simulink model "hoppingControl"  (R2018b)
settings: Solver=FixedStepAuto  StartTime=0.0  StopTime=inf  RelTol=1e-3  EnableMultiTasking=on
libraries: dspstat3 x19, cm_custom x9, raspberrypilib x8, simulink_extras x3, peGeneralControl x3, can_bus_multi x2, simulink x1, embdlinuxlib x1
(part 2 of 3)

== matlab function hoppingControl/Joint Position Filter/MATLAB Function ==
  data: motor_pos input; bias output; set_offset input; corrected_pos output; safe output
function [bias,corrected_pos, safe] = correct_pos(motor_pos, set_offset)
persistent offset;
persistent safety;
if(isempty(safety))
    safety = -1;
end

if(isempty(offset))
    offset = [0; 0; 0];
end


bias = offset;
if(set_offset~=0)
    offset = motor_pos(1:3);
    safety = 0;
elseif safety == 0
    safety = 1;
end
corrected_pos = motor_pos(1:3)-offset;
for i = 1:3
    if(corrected_pos(i)>180)
        corrected_pos(i) = corrected_pos(i) - 360;
    end

    if(corrected_pos(i)<-180)
        corrected_pos(i) = corrected_pos(i) + 360;
    end
    corrected_pos(i) = corrected_pos(i)+90;
    if corrected_pos(i)>90
        corrected_pos(i) = 90;
    end
end





safe = safety;
end

== matlab function hoppingControl/state estimation/MATLAB Function ==
  data: velInc input; vel output; angVelInc input; angVel input; viconPos input; viconOrient input; velLambda input; orientLambda input; orient output; realAngVel output; vVel output; vOrient output size=[1 4]; viconTime input; orientReset input; vPos output
function [vel,orient,realAngVel,vVel,vOrient,vPos] = sensorFusion(velInc, angVelInc, angVel, viconPos, viconOrient, velLambda, ...
                                                                  orientLambda,viconTime, orientReset)
persistent lastOrient;
if isempty(lastOrient)
    lastOrient = quaternion(1,0,0,0);
end
persistent lastOrientTime;
if isempty(lastOrientTime)
    lastOrientTime = 0;
end
persistent lastViconQuat;
if isempty(lastViconQuat)
    lastViconQuat = quaternion(1,0,0,0);
end

imu2vicon = [0  0 -1; % rotation matrix of robot frame in vicon to imu frame
            -1  0  0;
             0  1  0];
quatInc = compact(quaternion((imu2vicon*angVelInc)','rotvec'));
if quatInc(1)<0
    quatInc = -quatInc;
end
quatInc = quaternion(quatInc);
temp = compact(lastOrient * quatInc);
if temp(1)<0
    temp = -temp;
end
lastOrient = quaternion(temp);
if abs(viconTime-lastOrientTime)>=0.01
    viconQuat = compact(quaternion(viconOrient','euler','XYZ','frame'));
    if viconQuat(1)<0
        viconQuat = -viconQuat;
    end
    viconQuat = quaternion(viconQuat);
    errorQuat = viconQuat*conj(lastOrient);
    errorQuat = compact(errorQuat);
    if errorQuat(1)<0
        errorQuat = -errorQuat;
    end
    errorAngle = asin(norm(errorQuat(2:4)))*2;
    correctAngle = orientLambda*errorAngle;
    correctQuat = compact(quaternion(correctAngle*errorQuat(2:4)/norm(errorQuat(2:4)),'rotvec'));
    if correctQuat(1)<0
        correctQuat = -correctQuat;
    end
    correctQuat = quaternion(correctQuat);
    lastOrient = (correctQuat)*lastOrient;
    lastOrientTime = viconTime;
    lastViconQuat = viconQuat;
end

persistent lastVel;
if isempty(lastVel)
    lastVel = [0;0;0];
end
persistent lastViconVel;
if isempty(lastViconVel)
    lastViconVel = [0;0;0];
end
persistent lastPos;
if isempty(lastPos)
    lastPos = [0;0;0];
end
persistent lastViconVel2;
if isempty(lastViconVel2)
    lastViconVel2 = [0;0;0];
end
persistent lastPos2;
if isempty(lastPos2)
    lastPos2 = [0;0;0];
end
persistent lastVelTime
if isempty(lastVelTime)
    lastVelTime = 0;
end
lastVel = lastVel - quat2rotm(lastOrient)*imu2vicon*velInc - [0;0;9.81]*0.002;
if abs(viconTime - lastVelTime)>=0.01
    pos = viconPos +  quat2rotm(lastViconQuat)*[-0.01388;0.02222;-0.1656]; % robot center from vicon object center in vicon frame
    lastViconVel = (pos - lastPos)/(viconTime-lastVelTime);
    lastPos = pos;
    
    pos2 = viconPos +  quat2rotm(lastViconQuat)*[-0.0291;0.02197;-0.0568]; % imu from vicon object center in vicon frame
    lastViconVel2 = (pos2 - lastPos2)/(viconTime-lastVelTime);
    lastPos2 = pos2;
    lastVel = (1-velLambda)*lastVel+velLambda*lastViconVel2;
    lastVelTime = viconTime;
end
realAngVel = quat2rotm(lastOrient)*imu2vicon*angVel;
vel = lastVel-cross(realAngVel,quat2rotm(lastOrient)*[-0.01525;-0.0025;0.1088]); % z: 109.1mm - 0.3mm, off center of IMU % imu from robot center
% vel = viconPos-cross(realAngVel,quat2rotm(lastOrient)*[-0.01525;0;0.1634-0.035]);
orient = compact(lastOrient);
vVel = lastViconVel;
vOrient = compact(lastViconQuat);
if orientReset == 1
    lastOrient = lastViconQuat;
    lastVel = lastViconVel2;
end
vPos = lastPos2;

end

== matlab function hoppingControl/Motor Driver/MATLAB Function4 ==
  data: curr input; propCmd input; WingSafety input; current output; propeller_mode output; pos input; upperLim input; lowerLim input; buffer input; offsetSafety input; maxCurrent input; balanceSafety input; balanceReset input; propeller_curr output; propCurrMax input; propDutyMax input; propeller_duty output
function [current,propeller_mode,propeller_curr,propeller_duty] = check(curr,propCmd, WingSafety, pos,upperLim, lowerLim,buffer, offsetSafety, ...
                                                                        maxCurrent, balanceSafety, balanceReset, propCurrMax, propDutyMax)
persistent balanceSafe;

if isempty(balanceSafe)
    balanceSafe = 1;
end
if balanceSafety == 0 
    balanceSafe = 0;
end
if balanceReset == 1
    balanceSafe = 1;
end

current = curr;
propeller_mode = propCmd(1);
propeller_curr = propCmd(2:4);
propeller_duty = propCmd(2:4);
for i = 1:3
    if pos(i)>upperLim-buffer && current(i)>0
        current(i) = 0;
    elseif pos(i)<lowerLim+buffer && current(i)<0
        current(i) = 0;
    end
    if abs(current(i))>maxCurrent
        current = current/abs(current(i))*maxCurrent;
        
    end
    if propeller_curr(i)>propCurrMax
        propeller_curr(i) = propCurrMax;
    end
    if propeller_curr(i)<1
        propeller_curr(i) = 1;
    end
    if propeller_duty(i)>propDutyMax
        propeller_duty(i) = propDutyMax;
    end
    if propeller_duty(i)<0.12
        propeller_duty(i) = 0.12;
    end
end
%%P = pitchSafe;

if WingSafety == 0
    propeller_mode = 4;
    propeller_curr = [1;1;1];
    propeller_duty = [0;0;0];
end
if offsetSafety==-1 || balanceSafe ~= 1 || balanceReset == 1
    current = [0;0;0];
    propeller_mode = 4;
    propeller_curr = [0;0;0];
    propeller_duty = [0;0;0];
end
if offsetSafety == 0
    current = [0.3;0.3;0.3];
    propeller_mode = 4;
    propeller_curr = [0;0;0];
    propeller_duty = [0;0;0];
end


end

== matlab function hoppingControl/state estimation/MATLAB Function2 ==
  data: estimate_pAng output; quat_orient output; ang_vel output; estimate_vel output; imu_accel input; estimate_pos output; mapped_vicon_pos output; imu_gyro input; foot_pos input; foot_vel input; accel_weight input; orient_reset input; state input; bound input; debug output; arm_length input; vicon_flag input; orient_lambda input; vel_lambda input; vicon_pos input; vicon_orient input; vicon_time input
function [estimate_pAng,quat_orient,ang_vel,estimate_vel,estimate_pos,mapped_vicon_pos,debug] = com_filter(imu_accel,imu_gyro,foot_pos,foot_vel,accel_weight, ...
                                                                                   orient_reset,state,bound,arm_length, ...
                                                                                   vicon_flag,orient_lambda,vel_lambda, ...
                                                                                   vicon_pos,vicon_orient,vicon_time)
%% persistent initialize
persistent pAng
persistent state_count
persistent last_state
persistent stance_flag
persistent last_orient
persistent last_foot_vel
persistent last_foot_pos
persistent flight_vel
persistent last_pos
persistent last_vicon_time
persistent last_vicon_quat
persistent last_vicon_pos
persistent last_correcting_quat

if isempty(pAng)
    pAng = 0;
end
if isempty(state_count)
    state_count = 0;
end
if isempty(last_state)
    last_state = 1;
end
if isempty(stance_flag)
    stance_flag = 0;
end
if isempty(last_orient)
    last_orient = quaternion(1,0,0,0);
end
if isempty(last_foot_vel)
    last_foot_vel = zeros(10,3);
end
if isempty(last_foot_pos)
    last_foot_pos = zeros(10,3);
end
if isempty(flight_vel)
    flight_vel = [0;0;0];
end
if isempty(last_pos)
    last_pos = [0;0;0];
end
if isempty(last_vicon_time)
    last_vicon_time = 0;
end
if isempty(last_vicon_quat)
    last_vicon_quat = quaternion(1,0,0,0);
end
if isempty(last_vicon_pos)
    last_vicon_pos = [0;0;0];
end
if isempty(last_correcting_quat)
    last_correcting_quat = quaternion(1,0,0,0);
end

imu2vicon = [0  0 -1; % rotation matrix of robot frame in vicon to imu frame
            -1  0  0;
             0  1  0];
robot2vicon = [0 1  0;
               1 0  0;
               0 0 -1];
time_step = 0.002;
           
%% imu signal process
if isnan(imu_accel(1))
    last_pos = [100;100;100];
    imu_accel(1) = 0;
end
if isnan(imu_accel(2))
    last_pos = [100;100;100];
    imu_accel(2) = 0;
end
if isnan(imu_accel(3))
    last_pos = [100;100;100];
    imu_accel(3) = 0;
end
if isnan(imu_gyro(1))
    last_pos = [100;100;100];
    imu_gyro(1) = 0;
end
if isnan(imu_gyro(2))
    last_pos = [100;100;100];
    imu_gyro(1) = 0;
end
if isnan(imu_gyro(3))
    last_pos = [100;100;100];
    imu_gyro(1) = 0;
end

gyro_inc = imu2vicon*imu_gyro*time_step;
gyro_pAngInc = gyro_inc(1);
% gyro_pAngInc = imu_gyro(3)*time_step;
imu_accel = imu2vicon*imu_accel;
imu_accel_global = imu_accel;
imu_accel = imu_accel/norm(imu_accel);
accel_pAng = atan(imu_accel(2)/imu_accel(3));
pAng = (pAng+gyro_pAngInc);

quat_gyro_inc = compact(quaternion((gyro_inc)','rotvec'));
if quat_gyro_inc(1)<0
    quat_gyro_inc = -quat_gyro_inc;
end
quat_gyro_inc = quaternion(quat_gyro_inc);
temp = compact(last_orient*quat_gyro_inc);
if temp(1)<0
    temp = -temp;
end
last_orient = quaternion(temp); 

%% orient estimate
if state == 2 && last_state == 1
    stance_flag = 1;
    state_count = 0;
elseif state == 1 && last_state == 2
    stance_flag = 0;
    state_count = 0;
end

if stance_flag == 1
    if state_count>bound(1) && state_count<bound(2)
        pAng = (pAng+gyro_pAngInc)*(1-accel_weight)+accel_pAng*accel_weight;        
        correcting_accel = cross([0;0;1],-imu_accel);
        correcting_accel_ang = accel_weight*asin(norm(correcting_accel));
        temp = sin(correcting_accel_ang/2)*correcting_accel;
        correcting_quat = compact(quaternion(cos(correcting_accel_ang/2),temp(1),temp(2),temp(3)));
        if correcting_quat(1)<0
            correcting_quat = -correcting_quat;
        end
        correcting_quat = quaternion(correcting_quat);
        temp = compact(last_orient*correcting_quat);
        if temp(1)<0
            temp = -temp;
        end
        last_orient = quaternion(temp);
    end
    state_count = state_count+1;
end
hover_flag = 0;
if state == 99 && orient_reset == 0
    if state_count>2*500 && abs(norm(imu_accel_global)-1)<0.1 % assume flight phase duration > 2s is hovering when initialize
        hover_flag = 1;
        pAng = (pAng+gyro_pAngInc)*(1-accel_weight)+accel_pAng*accel_weight;        
        correcting_accel = cross([0;0;1],-imu_accel);
        correcting_accel_ang = accel_weight*asin(norm(correcting_accel));
        temp = sin(correcting_accel_ang/2)*correcting_accel;
        correcting_quat = compact(quaternion(cos(correcting_accel_ang/2),temp(1),temp(2),temp(3)));
        if correcting_quat(1)<0
            correcting_quat = -correcting_quat;
        end
        correcting_quat = quaternion(correcting_quat);
        temp = compact(last_orient*correcting_quat);
        if temp(1)<0
            temp = -temp;
        end
        last_orient = quaternion(temp);
    end
    state_count = state_count+1;
end

%%% vicon
if abs(vicon_time-last_vicon_time)>=0.01 && vicon_flag == 1
    vicon_quat = compact(quaternion(vicon_orient','euler','XYZ','frame'));
    if vicon_quat(1)<0
        vicon_quat = -vicon_quat;
    end
    vicon_quat = quaternion(vicon_quat);
    error_quat = vicon_quat*conj(last_orient);
    error_quat = compact(error_quat);
    if error_quat(1)<0
        error_quat = -error_quat;
    end
    error_angle = asin(norm(error_quat(2:4)))*2;
    correct_angle = orient_lambda*error_angle;
    correct_quat = compact(quaternion(correct_angle*error_quat(2:4)/norm(error_quat(2:4)),'rotvec'));
    if correct_quat(1)<0
        correct_quat = -correct_quat;
    end
    correct_quat = quaternion(correct_quat);
    temp = compact((correct_quat)*last_orient);
    if temp(1)<0
        temp = -temp;
    end
    last_orient = quaternion(temp);
    last_vicon_quat = vicon_quat;
end

ang_vel = quat2rotm(last_orient)*imu2vicon*imu_gyro;

%% vel estimate
for i = 1:length(last_foot_pos)
    if i <length(last_foot_pos)
        last_foot_vel(i,:) = last_foot_vel(i+1,:);
        last_foot_pos(i,:) = last_foot_pos(i+1,:);
    elseif i==length(last_foot_pos)
        last_foot_vel(i,:) = foot_vel;
        last_foot_pos(i,:) = foot_pos;
    end
end
avg_foot_vel = mean(last_foot_vel);
avg_foot_pos = mean(last_foot_pos);
robot_rotm = quat2rotm(last_orient);
if last_state == 2 && state == 1
    flight_vel = robot_rotm*(robot2vicon*-avg_foot_vel') + robot_rotm*(cross(ang_vel,robot2vicon*-avg_foot_pos'));
end

persistent viconVel
if isempty(viconVel)
    viconVel = [0;0;0];
end

if last_state == 1
    estimate_vel = flight_vel;
elseif last_state == 2
    estimate_vel = robot_rotm*(robot2vicon*-foot_vel) + robot_rotm*(cross(ang_vel,robot2vicon*-foot_pos));
else
    estimate_vel = [0;0;0];
end
estimate_vel(3)= 0;

if orient_reset == 1
    pAng = accel_pAng;
    rotv_accel = cross(-imu_accel,[0;0;1]);
    rotv_accel_ang = asin(norm(rotv_accel)/norm(imu_accel));
    temp = sin(rotv_accel_ang/2)*rotv_accel;
    quat_accel = compact(quaternion(cos(rotv_accel_ang/2),temp(1),temp(2),temp(3)));
    if quat_accel(1)<0
        quat_accel = -quat_accel;
    end
    
    last_orient = quaternion(quat_accel);
    
    if vicon_flag == 1
        last_orient = last_vicon_quat;
    end
    flight_vel = [0;0;0];
    estimate_vel = [0;0;0];
%     last_pos = [arm_length;0;0];
    last_pos = [0;0;0];
    state_count = 0;
end

%% output
estimate_pAng = pAng;
quat_orient = compact(last_orient);
estimate_pos = last_pos + estimate_vel*time_step;
% if abs(vicon_time-last_vicon_time)>=0.01
%     pos = vicon_pos +  quat2rotm(last_vicon_quat)*[-0.01388;0.02222;-0.1656];
%     vicon_vel = (pos-last_vicon_pos)/(vicon_time-last_vicon_time);
%     flight_vel = flight_vel*(1-vel_lambda)+vicon_vel*vel_lambda;
%     lin_vel_estimation = lin_vel_estimation*(1-vel_lambda)+vicon_vel*vel_lambda;
%     last_vicon_time = vicon_time;
%     last_vicon_pos = pos;
%     viconVel = vicon_vel;
% end
if abs(vicon_time-last_vicon_time)>=0.01 && vicon_flag == 1
    pos = vicon_pos +  quat2rotm(last_vicon_quat)*[-0.01388;0.02222;-0.1656];
    estimate_pos = estimate_pos*(1-vel_lambda)+last_vicon_pos*vel_lambda;
    last_vicon_time = vicon_time;
    last_vicon_pos = pos;
end
mapped_vicon_pos = last_vicon_pos;
    
debug = [imu_accel;hover_flag];

last_state = state;
last_pos = estimate_pos;

== matlab function hoppingControl/state estimation/MATLAB Function1 ==
  data: velInc input; imu_gyro input; foot_pos input; foot_vel input; orient_reset input; arm_length input; pAng input; new_vel output; imu_vel output; estimate_vel output; new_orient output; new_realAngVel output; new_vPos output; ePos output; debug output; state input; vel_weight input
function [new_vel,imu_vel,estimate_vel,new_orient,new_realAngVel,new_vPos,ePos,debug]  = fcn(velInc,imu_gyro,foot_pos,foot_vel,orient_reset, ...
                                                                                        arm_length,pAng,state,vel_weight)
persistent lastPos;
persistent lastP;
persistent lastH;
persistent lastVel;
persistent flightVel;
persistent orient;
persistent last_state;
persistent lastFootVel;
persistent lastFootPos;
persistent hAng_offset;
persistent hAng;
persistent rev_count;
if isempty(lastPos)
    lastPos = [0;0;0];
end
if isempty(lastP)
    lastP = 0;
end
if isempty(lastH)
    lastH = 0;
end
if isempty(lastVel)
    lastVel = [0;0;0];
end
if isempty(flightVel)
    flightVel = [0;0;0];
end
if isempty(last_state)
    last_state = 0;
end
if isempty(orient)
    orient = quaternion(1,0,0,0);
end
if isempty(lastFootVel)
    lastFootVel = zeros(10,3);
end
if isempty(lastFootPos)
    lastFootPos = zeros(10,3);
end
if isempty(hAng_offset)
    hAng_offset = 0;
end
if isempty(hAng)
    hAng = 0;
end
if isempty(rev_count)
    rev_count = 0;
end

time_step = 0.002;

if pAng > 180
    pAng = pAng - 360;
elseif pAng < -180
    pAng = pAng + 360;
end
if pAng-lastP>180
    pVel = (pAng-lastP-360)/time_step;
elseif pAng-lastP<-180
    pVel = (pAng-lastP+360)/time_step;
else
    pVel = (pAng-lastP)/time_step;
end
lastP = pAng;
pAng = pAng*pi/180;
pVel = pVel*pi/180;

% map imu's angVel as hAng
hAng_inc = imu_gyro(2)*time_step/cos(pAng);
hAng = hAng+hAng_inc;
if hAng > 2*pi
    hAng = hAng - 2*pi;
    rev_count = rev_count+1;
elseif hAng < 0
    hAng = hAng + 2*pi;
    rev_count = rev_count-1;
end
if hAng-lastH>pi
    hVel = (hAng-lastH-2*pi)/time_step;
elseif hAng-lastH<-pi
    hVel = (hAng-lastH+2*pi)/time_step;
else 
    hVel = (hAng-lastH)/time_step;
end
lastH = hAng;
% hAng = hAng*pi/180;
% hVel = hVel*pi/180;

x = arm_length*cos((hAng-hAng_offset));
y = arm_length*sin((hAng-hAng_offset));

pRotm = [1 0 0;
         0 cos(pAng) -sin(pAng);
         0 sin(pAng) cos(pAng)]; % pitch is robot's y, vicon's x
hRotm = [cos(hAng-hAng_offset) -sin(hAng-hAng_offset) 0;
         sin(hAng-hAng_offset) cos(hAng-hAng_offset) 0;
         0 0 1]; % horizontal is robot's -z, vicon's z
% robotRotm = hRotm*pRotm;
robotRotm = pRotm;
temp = compact(quaternion(robotRotm','rotmat','frame'));
if temp(1)<0
    temp = -temp;
end
orient = quaternion(temp);

imu2vicon = [0  0 -1; % rotation matrix of robot frame in vicon to imu frame
            -1  0  0;
             0  1  0];
robot2vicon = [0 1  0;
               1 0  0;
               0 0 -1];
% realAngVel = hRotm*[pVel;0;0]+[0;0;hVel];
realAngVel = [pVel;0;0];
lastVel = lastVel-quat2rotm(orient)*imu2vicon*velInc-[0;0;9.81]*0.002;

% estimator
for i = 1:10
    if i <10
        lastFootVel(i,:) = lastFootVel(i+1,:);
        lastFootPos(i,:) = lastFootPos(i+1,:);
    elseif i==10
        lastFootVel(i,:) = foot_vel;
        lastFootPos(i,:) = foot_pos;
    end
end
avgFootVel = mean(lastFootVel);
avgFootPos = mean(lastFootPos);
lin_vel_estimation = robotRotm*(robot2vicon*-avgFootVel') + robotRotm*(cross(realAngVel,robot2vicon*-avgFootPos'));
if last_state == 2 && state == 1
    flightVel = lin_vel_estimation;
end

if last_state == 1
    estimate_vel = flightVel;
elseif last_state == 2
    estimate_vel = lin_vel_estimation;
else
    estimate_vel = [0;0;0];
end

lastVel = lastVel*(1-vel_weight)+estimate_vel*vel_weight;
lastVel = lastVel-cross(realAngVel,quat2rotm(orient)*[-0.01525;-0.0025;0.1088]);
imu_vel = lastVel;

if orient_reset == 1
    lastVel = [0;0;0];
    flightVel = [0;0;0];
    imu_vel = [0;0;0];
    estimate_vel = [0;0;0];
    lastPos = [0;0;0];
    hAng = 0;
    rev_count = 0;
    hAng_offset = hAng;
end

new_orient = compact(orient);

new_realAngVel = [pVel;0;0];
new_vel = [0;hVel;0];
new_vPos = [0;arm_length*(hAng-hAng_offset)+2*pi*rev_count;0];
% new_realAngVel = realAngVel;
% new_vPos = [x;y;0];
% new_vel = hVel*cross([0;0;1],new_vPos/norm(new_vPos));

ePos = lastPos + estimate_vel*time_step;
ePos(3) = 0;

debug = [pAng;hAng-hAng_offset;pVel;hVel];

lastPos = ePos;
last_state = state;

== matlab function hoppingControl/MATLAB Function ==
  data: Zoffset input; torque output; X input; xdot input; joint input; jointVel input; vel input; quat input; angVel input; robotPos input; J input; l0 input; k input; b input; m input; h input; desiredPos input; stepperLim input; Kp input; Kv input; Kr input; Khp input; Khd input; Kpp input; Kpd input; hipTorqueLim input; Kpos input; posVelLim input; propKp input; propKd input; Kpj input; Kdj input; flip input; clock input; balanceSafety output; debug output; desirePropCurr output; flipping output
function [torque,balanceSafety,debug,desirePropCurr,flipping] = virtual_spring(Zoffset,X,xdot,joint,jointVel,vel,quat,angVel,robotPos, ...
                                                                               J,l0,k,b,m,h,desiredPos,stepperLim,Kp,Kv,Kr,Khp,Khd,Kpp,Kpd, ...
                                                                               hipTorqueLim, Kpos, posVelLim, propKp, propKd, Kpj, Kdj, flip, clock)
persistent state;
if isempty(state)
    state = 1;
end
persistent state_safety;
if isempty(state_safety)
    state_safety = 0;
end
persistent lastFlip;
if isempty(lastFlip)
    lastFlip  = 0;
end
persistent afterFlip;
if isempty(afterFlip)
    afterFlip  = 0;
end
persistent time
if isempty(time)
    time = clock;
end
persistent wing_Override;
if isempty(wing_Override)
    wing_Override  = 0;
end
propDirection=[0;0];

robot2vicon = [ 0 1 0; 1 0 0 ;0 0 -1];
quat = quaternion([quat(1) quat(2) quat(3) quat(4)]);
vicon2world = quat2rotm(quat);

rAngVel = robot2vicon'*vicon2world'*angVel;
%%% for 3D
if desiredPos(3) == 0
    desiredVel = Kpos*(desiredPos-robotPos);
else
    desiredVel = [0;desiredPos(2);0];
end
% if afterFlip > 0
%     desiredVel = [0;0;0];
% end
if norm(desiredPos-robotPos)>1.3
%     state = 1000;
end
% if robotPos(3)>0.85 && robotPos(3)<0.95
%     afterFlip = 3;
% end

%%% for 2D
% with vicon
% robot_r = -atan((2*quat(4)*quat(1) - 2*quat(2)*quat(3))/(1 - 2*quat(3)*quat(3) - 2*quat(4)*quat(4))); % rotate robot Z-axis
% if robotPos(1)>0
%     robot_r = robot_r+pi;
% end
% if robot_r<0
%     robot_r = robot_r+2*pi;
% end
% if desiredPos(1) == 0
%     angle_diff = desiredPos(2)*pi/180-robot_r;
%     if abs(angle_diff)>pi
%         angle_diff = -angle_diff+sign(angle_diff)*pi;
%     end
%     tempVel = Kpos*(angle_diff);
% elseif desiredPos(1) == 1
%     tempVel = desiredPos(2);
% else
%     tempVel = 0;
% end
% desiredVel = [tempVel*sin(robot_r);tempVel*cos(robot_r);0];
% % % % % eulerZYX = quat2eul(quat); % euler Z from -180 to 180
% % % % % eulerZ = eulerZYX(1);
% % % % % angle_diff = 0;
% % % % % if desiredPos(1) == 0
% % % % %     angle_diff = desiredPos(2)*pi/180-eulerZ;
% % % % %     if abs(angle_diff)>pi
% % % % % %         angle_diff = -angle_diff+sign(angle_diff)*pi;
% % % % %         angle_diff = -pi*sign(angle_diff)+(angle_diff-pi*sign(angle_diff));
% % % % %     end
% % % % %     tempVel = Kpos*(angle_diff);
% % % % % elseif desiredPos(1) == 1
% % % % %     tempVel = desiredPos(2);
% % % % % else
% % % % %     tempVel = 0;
% % % % % end
% % % % % desiredVel = [0;-tempVel;0];
% % % % % desiredVel = vicon2world*desiredVel;
% with encoder
% % % hAng = robotPos(2);
% % % angle_diff = desiredPos(2)*pi/180-hAng;
% % % desiredVel = [0;Kpos*angle_diff;0];
%%% with imu, 3D code
% % % eulerZYX = quat2eul(quat); % euler Z from -180 to 180
% % % eulerZ = eulerZYX(1);
% % % % map eulerZ to: from 0 to 360
% % % if eulerZ<0
% % %     eulerZ = eulerZ+2*pi;
% % % end
% % % angle_diff = 0;
% % % if desiredPos(1) == 0
% % %     angle_diff = desiredPos(2)*pi/180-eulerZ;
% % %     if angle_diff<=-pi
% % %         angle_diff = angle_diff+2*pi;
% % %     elseif angle_diff>=pi
% % %         angle_diff = angle_diff-2*pi;
% % %     end
% % %     tempVel = Kpos*angle_diff;
% % % elseif desiredPos(1) == 1
% % %     tempVel = desiredPos(2);
% % % else
% % %     tempVel = 0;
% % % end
% % % desiredVel = [tempVel*sin(-eulerZ);tempVel*cos(-eulerZ);0];

% without vicon
% robotPos = robotPos*pi/180;
% if desiredPos(1) == 0
%     angle_diff = desiredPos(3)*pi/180-robotPos(3);
%     if abs(angle_diff)>pi
%         angle_diff = -pi*sign(angle_diff)+(angle_diff-pi*sign(angle_diff));
%     end
%     tempVel = Kpos*(angle_diff);
% elseif desiredPos(1) == 1
%     tempVel = desiredPos(2);
% else
%     tempVel = 0;
if norm(desiredVel)>posVelLim
    desiredVel = desiredVel/norm(desiredVel)*posVelLim;
end

x = X-[0;0;Zoffset];
l = norm(x);
unitSpring = x/l;
springVel = dot(xdot,unitSpring)*unitSpring;
groundHeight = dot(vicon2world*robot2vicon*x,[0;0;-1]);
energy = 1/2*m*dot(springVel,springVel)+ 1/2*k*(l0-l)^2 + m*9.81*(groundHeight);
target = m*9.81*(l0+h)+1/2*m*dot(desiredVel,desiredVel);
error = target-energy;
force = -k*(l-l0);
% Propellers
prop_mode = 4;
wing_a = 1;
wing_b = 1;
wing_c = 1;

flipping = 0;
balanceSafety = 1;
% if  acos(dot([0;0;1],vicon2world*[0;0;1])) > 60*pi/180 || l<l0-0.15 || (state_safety > 1000 && prop_mode == 5)% || robot_p > 60*pi/180
%     balanceSafety = 0;
% end
if state < 3 || state > 7
    if acos(dot([0;0;1],vicon2world*[0;0;1])) > 30*pi/180
        state = 1001;
    elseif (state_safety > 400 && prop_mode == 5)
        state = 1002;
    elseif abs(l-l0)>0.15 && flip ~= 1
        state = 1003;
%     elseif robotPos(3)<0.4
%         state = 1004;
%     elseif norm(desiredPos(1)-robotPos(1))>1 || norm(desiredPos(2)-robotPos(2))>1
%         state = 1005;
    end
end
footForce = [0;0;0];
worldUp = robot2vicon'*vicon2world'*[0;0;1];
robotTilt = cross(worldUp,[0;0;-1]); %% world up is in the direction ofnote negative z in robot frame
if norm(robotTilt)>0.01
    robotTilt = robotTilt/norm(robotTilt)*acos(dot(worldUp,[0;0;-1]));
end
% for flipping, angle between wing_b vector and world up, init at 90deg, towards 0
wing_bAng = cross(worldUp,[0;-1;0]);
if norm(wing_bAng)>0.01
    wing_bAng = wing_bAng/norm(wing_bAng)*acos(dot(worldUp,[0;-1;0]));
end
% wing_aAng = cross(worldUp,[0;-1;0]);
% if norm(wing_bAng)>0.01
%     wing_aAng = wing_aAng/norm(wing_aAng)*acos(dot(worldUp,[0;-1;0]));
% end
% wing_cAng = cross(worldUp,[0;-1;0]);
% if norm(wing_cAng)>0.01
%     wing_cAng = wing_cAng/norm(wing_cAng)*acos(dot(worldUp,[0;-1;0]));
% end
if state == 1 % flight phase
%%calculate foot pos in world frame centered at robot origin

    ground = 0;
    targetFootPos = Kv*[vel(1);vel(2);0] - Kr*[desiredVel(1); desiredVel(2); 0];
    normTarget = norm(targetFootPos);
%     if afterFlip > 0
%         stepperLim = 0.1;
%     end
    if normTarget>stepperLim
        targetFootPos = targetFootPos/normTarget*0.1;
    end
    targetFootPos(3) = - sqrt(l0^2-normTarget^2);
    normTarget = l0;
    targetFootPos = robot2vicon'*vicon2world'*targetFootPos;
    sideForce = Khp*(targetFootPos-x)-Khd*(xdot-cross(rAngVel,x));
    sideForce = sideForce - dot(sideForce,unitSpring)*unitSpring;
    springForce = force*unitSpring-b*springVel;
    footForce = sideForce+springForce;
    torque = J'\footForce;
    state_safety = state_safety+1;
    if flip == 0
        lastFlip = 0;
    end 
    if l<l0-0.02 && ...
       norm(robotTilt)<30*pi/180 && ... 
       flip == 1 && ...
       lastFlip == 0 && ...
       norm([rAngVel(1) rAngVel(2)])<5 && ...
       (norm([targetFootPos(1) targetFootPos(2)]) < 0.023 && norm([x(1) x(2)]) < 0.023) && ...
       norm(desiredPos(2)-robotPos(2))<0.25 && ...
       norm(desiredPos(1)-robotPos(1))<0.25
        state = 3;
        lastFlip = flip;
        time = clock;
        state_safety = 0;
    elseif l<l0-0.02
        state = 2;
        state_safety = 0;
    end
%     if (abs(robot_p)>30*pi/180 || abs(rAngVel(2))>6) && wing_Override == 0
%         state = 8;
%         state_safety = 0;
%         time = clock;
%     end
    
    % propeller control
    % 2D
%     if robot_p<-10*pi/180 || rAngVel(2)<-5
%         prop_mode = 5;
% %         wing_c = 1/50*round((abs(robot_p)*propKp-angVel(1)*propKd));
%         wing_a = 0.12;
%         wing_b = 0.12;
%         wing_c = 0.3*propKp;
%         if robot_p<-15*pi/180
%             wing_c = 0.5*propKd;
% %             if robot_p<-30*pi/180
% %                 wing_c = 0.7*propKd;
% %             end
%         end
%     elseif robot_p>10*pi/180 ||rAngVel(2)>5
%         prop_mode = 5;
%         wing_a = 0.3*propKp;
%         wing_b = 0.12;
%         wing_c = 0.12;
% %         wing_a = 1/50*round((abs(robot_p)*propKp-angVel(1)*propKd));
%         if robot_p>15*pi/180
%             wing_a = 0.5*propKd;
% %             if robot_p>30*pi/180
% %                 wing_a = 0.7*propKd;
% %             end
%         end
%     else
% %     if robot_p<-10*pi/180
% %         prop_mode = 4;
% %         wing_c = abs(robot_p)*propKp-angVel(1)*propKd;
% %         wing_a = 1;
% %     elseif robot_p>10*pi/180
% %         prop_mode = 4;
% %         wing_c = 1;
% %         wing_a = abs(robot_p)*propKp-angVel(1)*propKd;
% %     else
%         prop_mode = 4;
%         wing_a = 1;
%         wing_b = 1;
%         wing_c = 1;
%     end
    
    % 3D
    if norm(robotTilt)>3*pi/180        
        if robotTilt>25*pi/180
            propKp = 0.5;
        end
        propDuty = propKp*robotTilt + propKd*(rAngVel);
%         if norm(robotTilt)>20*pi/180
%             propDuty = 1*robotTilt + propKd*(rAngVel);
%         end
        if norm(propDuty)>0.5
            propDuty = propDuty / norm(propDuty)*0.5;
        end
        propDirection = cross(propDuty,[0;0;-1]);
        %  axis_b in local frame = [0;-1;0];
        prop_mode = 5;
        if acos(dot(propDirection/norm(propDirection),[0;-1;0])) <= 120*pi/180 % check near b
            if acos(dot(propDirection/norm(propDirection),[-sqrt(3)/2;0.5;0])) <= 120*pi/180 % check near a
                propInput = [-sqrt(3)/2 0; 0.5 -1]\[propDirection(1);propDirection(2)];
                wing_a = 0.12+propInput(1);
                wing_b = 0.12+propInput(2);
                wing_c = 0.12;
            elseif acos(dot(propDirection/norm(propDirection),[sqrt(3)/2;0.5;0])) <= 120*pi/180 % check near c
                propInput = [0 sqrt(3)/2; -1 0.5]\[propDirection(1);propDirection(2)];
                wing_a = 0.12;
                wing_b = 0.12+propInput(1);
                wing_c = 0.12+propInput(2);
            end
        else
            propInput = [-sqrt(3)/2 sqrt(3)/2; 0.5 0.5]\[propDirection(1);propDirection(2)];
            wing_a = 0.12+propInput(1);
            wing_b = 0.12;
            wing_c = 0.12+propInput(2);
        end
    else
        prop_mode = 4;
        wing_a = 1;
        wing_b = 1;
        wing_c = 1;
    end
    if afterFlip > 0
        if robotTilt>25*pi/180
            propKp = 0.2;
        end
        propDuty = (propKp*robotTilt + propKd*(rAngVel))/2;
        if norm(propDuty)>0.5
            propDuty = propDuty / norm(propDuty)*0.5;
        end
        propDirection = cross(propDuty,[0;0;1]);
        %  axis_b in local frame = [0;-1;0];
        prop_mode = 5;
        if acos(dot(propDirection/norm(propDirection),[0;-1;0])) <= 120*pi/180 % check near b
            if acos(dot(propDirection/norm(propDirection),[-sqrt(3)/2;0.5;0])) <= 120*pi/180 % check near a
                propInput = [-sqrt(3)/2 0; 0.5 -1]\[propDirection(1);propDirection(2)];
                wing_a = 0.32-propInput(1);
                wing_b = 0.32-propInput(2);
                wing_c = 0.32;
            elseif acos(dot(propDirection/norm(propDirection),[sqrt(3)/2;0.5;0])) <= 120*pi/180 % check near c
                propInput = [0 sqrt(3)/2; -1 0.5]\[propDirection(1);propDirection(2)];
                wing_a = 0.32;
                wing_b = 0.32-propInput(1);
                wing_c = 0.32-propInput(2);
            end
        else
            propInput = [-sqrt(3)/2 sqrt(3)/2; 0.5 0.5]\[propDirection(1);propDirection(2)];
            wing_a = 0.32-propInput(1);
            wing_b = 0.32;
            wing_c = 0.32-propInput(2);
        end
%         wing_a = 0.32;
%         wing_b = 0.32;
%         wing_c = 0.32;
    end

elseif state == 2 % stance phase
    ground = 10;
    springForce = force;
     if dot(xdot,unitSpring) > 0.1
        springForce = springForce + sign(dot(xdot,unitSpring))*Kp*error;
     end
     if springForce<0
        springForce = 0;
     end
    springForce = springForce*unitSpring;
%     worldUp = robot2vicon'*vicon2world'*[0;0;1];
%     robotTilt = cross(worldUp,[0;0;-1]); %% world up is in the direction ofnote negative z in robot frame
%     if norm(robotTilt)>0.01
%         robotTilt = robotTilt/norm(robotTilt)*acos(dot(worldUp,[0;0;-1]));
%     end
    %%else use small angle sine approximation
    hipTorque = Kpp*robotTilt + Kpd*(rAngVel);
    hipTorque = hipTorque-dot(hipTorque,unitSpring)*unitSpring;
    if afterFlip > 0
        hipTorqueLim = 1.5;
    end
    if norm(hipTorque)>hipTorqueLim
        hipTorque = hipTorque / norm(hipTorque)*hipTorqueLim;
    end
    sideForce = cross(hipTorque,x)/dot(x,x);
    footForce = springForce+sideForce;
    torque = J'\footForce;
    state_safety = state_safety+1;
    if l>l0
        state = 1;
        state_safety = 0;
        if afterFlip > 0
            afterFlip = afterFlip-1;
        end
    end
    
    % propeller control
%     if (abs(robot_p)>30*pi/180 || abs(rAngVel(2))>6) && wing_Override == 0
%         state = 8;
%         state_safety = 0;
%         time = clock;
%     end
    prop_mode = 4;
    wing_a = 1;
    wing_b = 1;
    wing_c = 1;
%     if afterFlip > 0
%     prop_mode = 5;
%     wing_a = 0.2;
%     wing_b = 0.2;
%     wing_c = 0.2;
%     end

elseif state == 3
    ground = 10;
    boo = 1;
    target = 1/2*k*0.251*0.25;
    error = target-energy;
    springForce = 0.5*force;
     if abs(dot(xdot,unitSpring)) > 0.1
        springForce = springForce + sign(dot(xdot,unitSpring))*Kp*error;
     end
     if springForce<0
        springForce = 0;
     end
    springForce = springForce*unitSpring;
%     hipTorque = (Kpp*[0;robot_p;0] + Kpd*([0;rAngVel(2);0]))/2;
    hipTorque = Kpp*robotTilt + Kpd*(rAngVel)/2;
    hipTorque = hipTorque-dot(hipTorque,unitSpring)*unitSpring;
    if norm(hipTorque)>hipTorqueLim
        hipTorque = hipTorque / norm(hipTorque)*hipTorqueLim;
    end
    sideForce = cross(hipTorque,x)/dot(x,x);
    footForce = springForce+sideForce;
    torque = J'\footForce;
    if l<l0-0.18
        state = 4;
        time = clock;
    elseif l>l0 || norm(robotTilt)<-170*pi
        state = 1030;
    end
    if abs(rAngVel(1))>4 || abs(rAngVel(2))>4 || abs(rAngVel(3))>4
        state = 1035;
        time = clock;
    end
    balanceSafety = 1;
    if norm(robotTilt)>5*pi/180
        balanceSafety = 0;
    end
    
elseif state == 4
    ground = 10;
    boo = 2;
    springForce = force;
    springForce = 120;
    springForce = springForce*unitSpring;
    prop_mode = 5;
    wing_a = 0.12;
    wing_b = 0.8;
    wing_c = 0.12;
    if rAngVel(2) > 0 %|| robot_y>3*pi/180
        wing_a = 0.12+propKd*abs(rAngVel(2));%+abs(robot_y)*0.5;
    elseif rAngVel(2) < 0 %|| robot_y<-3*pi/180
        wing_c = 0.12+propKd*abs(rAngVel(2));%+abs(robot_y)*0.5;
    end
    wing_a = min(max(0.12,wing_a),0.3);
    wing_c = min(max(0.12,wing_c),0.3);
%     hipTorque = [0;2;0];
    % for height test
    hipTorque = [0;0;0];
    hipTorque = hipTorque-dot(hipTorque,unitSpring)*unitSpring;
    sideForce = cross(hipTorque,x)/dot(x,x);
    footForce = springForce+sideForce;
    torque = J'\footForce;

    torque = torque/max(torque)*25*0.0561*5;
%     
    % for 2D
%     hipTorque = [0;2;0];
    % for 3D
    hipTorque = [-3;0;0];
%     hipTorque = [0;0;0];
    hipTorque = hipTorque-dot(hipTorque,unitSpring)*unitSpring;
    sideForce = cross(hipTorque,x)/dot(x,x);
    torque = torque+J'\sideForce;
%     if abs(rAngVel(2))>2.5 || abs(rAngVel(3))>4
%         state = 1045;
%         time = clock;
%     end
    if l>0.475
        state = 5;
        time = clock;
    elseif clock - time > 0.5
        state = 1040;
        time = clock;
    end
    balanceSafety = 1;
    flipping = 1;
    
elseif state == 5
%     if (norm(wing_bAng)<0*180/pi && norm(wing_bAng)>-90*pi/180)
        prop_mode = 5;
        wing_a = 0.12;
        wing_b = 0.4;
        wing_c = 0.12;
%     end
%     torque = Kpj*([-65*pi/180;-65*pi/180;-65*pi/180]-joint)-Kdj*jointVel;
    torque = Kpj*([45*pi/180;45*pi/180;45*pi/180]-joint)-Kdj*jointVel;
    for i = 1:3
        torque(i) = min(max(-5,torque(i)),5);
    end
    if norm(wing_bAng) < 20*pi/180
%         state = 5.5;
        time = clock;
    elseif clock-time>0.3
        state = 1050;
%         state = 1;
        time = clock;
    end
    balanceSafety = 1;
    flipping = 1;
    
elseif state == 5.5
%     if norm(wing_bAng) <= 22*pi/180% rAngVel(1)<11
        prop_mode = 5;
        wing_a = 0.12;
        wing_b = 0.12;
        wing_c = 0.12;
%     end
    torque = Kpj*([-65*pi/180;-65*pi/180;-65*pi/180]-joint)-Kdj*jointVel;
    for i = 1:3
        torque(i) = min(max(-5,torque(i)),5);
    end
    if norm(wing_bAng) > 20*pi/180
        state = 6;
        time = clock;
    elseif clock-time>0.5
        state = 1055;
        time = clock;
    end
    balanceSafety = 1;
    flipping = 1;
    
elseif state == 6
    prop_mode = 5;
    wing_a = 0.12;
    wing_b = 0.12;
    wing_c = 0.12;
    if norm(wing_bAng) > 60*pi/180
        wing_a = 0.5;
        wing_b = 0.12;
        wing_c = 0.5;
    end
    torque = Kpj*([-65*pi/180;-65*pi/180;-65*pi/180]-joint)-Kdj*jointVel;
    for i = 1:3
        torque(i) = min(max(-5,torque(i)),5);
    end
    if norm(wing_bAng) > 150*pi/180
        state = 6.5;
        time = clock;
    elseif clock-time>0.5
        state = 1060;
        time = clock;
    end
    balanceSafety = 1;
    flipping = 1;
    
elseif state == 6.5
    prop_mode = 5;
    wing_a = 0.5;
    wing_b = 0.12;
    wing_c = 0.5;
    if norm(wing_bAng) < 139*pi/180
        wing_a = 0.4;
        wing_b = 0.12;
        wing_c = 0.4;
    end
    if rAngVel(1)<3
        wing_a = 0.12;
        wing_b = 0.12;
        wing_c = 0.12;
    end
    torque = Kpj*([-65*pi/180;-65*pi/180;-65*pi/180]-joint)-Kdj*jointVel;
    for i = 1:3
        torque(i) = min(max(-5,torque(i)),5);
    end
    if norm(wing_bAng) < 120*pi/180
        state = 7;
        time = clock;
    elseif clock-time>0.5
        state = 1065;
        time = clock;
    end
    balanceSafety = 1;
    flipping = 1;
    
elseif state == 7
%     if  rAngVel(2)<-2%%||robot_p<-15*pi/180
%         props(2) = 30;
%     end
%     if robot_p>10*pi/180 ||(rAngVel(2)>2 && abs(robot_p)<15*pi/180)% || rAngVel(2)>5
%        prop_mode = 5;
%         wing_a = 0.7;
%         wing_b = 0.12;
%         wing_c = 0.12;
%     elseif robot_p <-10*pi/180 ||(rAngVel(2)<-2&&abs(robot_p)<15*pi/180)% || rAngVel(2)<-5
%        prop_mode = 5;
%         wing_a = 0.12;
%         wing_b = 0.12;
%         wing_c = 0.8;
%     end
%     if norm(robotTilt)>2*pi/180
%         propDuty = propKp*robotTilt + propKd*(rAngVel);
%         if norm(propDuty)>0.7
%             propDuty = propDuty / norm(propDuty)*0.7;
%         end
%         propDirection = cross(propDuty,[0;0;-1]);
%         %  axis_b in local frame = [-1;0;0];
%         prop_mode = 5;
%         if acos(dot(propDirection/norm(propDirection),[0;-1;0])) <= 120*pi/180 % check near b
%             if acos(dot(propDirection/norm(propDirection),[-sqrt(3)/2;0.5;0])) <= 120*pi/180 % check near a
%                 propInput = [-sqrt(3)/2 0; 0.5 -1]\[propDirection(1);propDirection(2)];
%                 wing_a = 0.12+propInput(1);
%                 wing_b = 0.12+propInput(2);
%                 wing_c = 0.12;
%             elseif acos(dot(propDirection/norm(propDirection),[sqrt(3)/2;0.5;0])) <= 120*pi/180 % check near c
%                 propInput = [0 sqrt(3)/2; -1 0.5]\[propDirection(1);propDirection(2)];
%                 wing_a = 0.12;
%                 wing_b = 0.12+propInput(1);
%                 wing_c = 0.12+propInput(2);
%             end
%         else
%             propInput = [-sqrt(3)/2 sqrt(3)/2; 0.5 0.5]\[propDirection(1);propDirection(2)];
%             wing_a = 0.12+propInput(1);
%             wing_b = 0.12;
%             wing_c = 0.12+propInput(2);
%         end
    prop_mode = 5;
    if rAngVel(2)>4 || norm(wing_bAng) >120*pi/180 ||(rAngVel(2)>1.5 && abs(90-norm(wing_bAng))<10*pi/180)
        wing_a = 0.45;
        wing_b = 0.12;
        wing_c = 0.45;
    elseif rAngVel(2)<-4 || norm(wing_bAng)<60*pi/180 ||(rAngVel(2)<-1.5 && abs(90-norm(wing_bAng))<10*pi/180)
        wing_a = 0.12;
        wing_b = 0.4;
        wing_c = 0.12;
    else
        wing_a = 0.12;
        wing_b = 0.12;
        wing_c = 0.12;
    end
%     torque = Kpj*([-65*pi/180;-65*pi/180;-65*pi/180]-joint)-Kdj*jointVel;
%     if robotPos(3)<0.8 || (clock-time)>0.15
        torque = Kpj*([30*pi/180;30*pi/180;30*pi/180]-joint)-Kdj*jointVel;
%     end
    for i = 1:3
       torque(i) = min(max(-5,torque(i)),5);
    end
    if joint(1)>30*pi/180 && joint(2)>30*pi/180 && joint(3)>30*pi/180
        state = 1;
        afterFlip = 3;
    end
    if clock-time>0.7
        state = 1070;
        time = clock;
    end    
    balanceSafety = 1;
       
elseif state == 8 % impact reduction mode
    torque = Kpj*([-65*pi/180;-65*pi/180;-65*pi/180]-joint)-Kdj*jointVel;
    for i = 1:3
        torque(i) = min(max(-5,torque(i)),5);
    end
    state_safety = state_safety+1;
    if clock - time > 0.1
        wing_Override = 200;
        state = 1;
        state_safety = 0;
        time = clock;
    end
    balanceSafety = 1;
    if acos(dot([0;0;1],vicon2world*[0;0;1])) > 60*pi/180
        balanceSafety = 0;
    end
else
    prop_mode = 4;
    wing_a = 0;
    wing_b = 0;
    wing_c = 0;
    torque = Kpj*([-20*pi/180;-20*pi/180;-20*pi/180]-joint)-Kdj*jointVel;
%     torque = [0;0;0];
    state_safety = state_safety+1;
    if state_safety>250
        state = 1;
        state_safety = 0;
        balanceSafety = 0;
    end
end
%     debug =[acos(dot(robot2vicon'*vicon2world'*[0;0;1],[0;0;-1]));ground];
%debug = l;

if prop_mode == 5
    wing_a = max(0.12,min(wing_a,0.5));
    wing_b = max(0.12,min(wing_b,0.5));
    wing_c = max(0.12,min(wing_c,0.5));
    if state >= 3 && state <= 5.5
        wing_a = max(0.12,min(wing_a,0.7));
        wing_b = max(0.12,min(wing_b,0.7));
        wing_c = max(0.12,min(wing_c,0.7));
    end
end

if wing_Override>0
    prop_mode = 5;
    wing_a = 0.7;
    wing_b = 0.7;
    wing_c = 0.7;
    wing_Override = wing_Override-1;
end
% desirePropCurr = [prop_mode; wing_a; wing_b; wing_c];
desirePropCurr = [prop_mode;footForce];

debug = [l desiredVel(1) desiredVel(2) ...
         rAngVel(1) rAngVel(2) rAngVel(3) ...
         vel(1) vel(2) ...
         state ...
         sqrt(vel(1)*vel(1)+vel(2)*vel(2))];
% debug = [desiredVel robotPos robot_ypr];
end
